simulink model "ysw3_46"  (R2014a)
settings: Solver=ode45  StartTime=0.0  StopTime=10.0  RelTol=1e-3
settings Model: Creator=Administrator  LastModifiedBy=Administrator

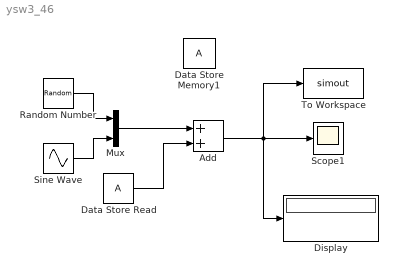
== system ysw3_46 ==
  Add : Sum
  Data Store Memory1 : DataStoreMemory  ReadBeforeWriteMsg=warning  WriteAfterWriteMsg=warning  WriteAfterReadMsg=warning  InitialValue=25  OutDataTypeStr=double
  Data Store Read : DataStoreRead
  Display : Display
  Mux : Mux  Inputs=2
  Random Number : RandomNumber  SampleTime=0.1
  Scope1 : Scope
      settings: TimeRange=10
  Sine Wave : Sin  SampleTime=0.1
  To Workspace : ToWorkspace  VariableName=simout  SaveFormat=Timeseries  SampleTime=-1
  wires:
  Random Number/1 -> Mux/1
  Sine Wave/1 -> Mux/2
  Mux/1 -> Add/1
  Data Store Read/1 -> Add/2
  Add/1 -> Display/1, Scope1/1, To Workspace/1
